simulink model "Sim_PIControl_PC"  (R2025b)
settings: Solver=VariableStepAuto  StartTime=0.0  StopTime=3  FixedStep=Ts  RelTol=1e-3
values from neighbouring files (symbols this model uses):
  Cf = Cf_values(k)    [Init_OSQP_PC.m]    (also in PC_PIControl.m = 1.2e-05)
  Ki_if = (sqrt(5) - 2)*Ki*wci^2    [PC_PIControl.m]
  Ki_vc = (sqrt(5) - 2)*Kv*wcv^2    [PC_PIControl.m]
  kP = ((2*pi*50.5) - (2*pi*49.5))/(2*10e3)    (= 0.000314159265359)    [PC_PIControl.m]
  Kp_if = (sqrt(2)*sqrt(sqrt(5) - 2))*Ki*wci    [PC_PIControl.m]
  Kp_vc = (sqrt(2)*sqrt(sqrt(5) - 2))*Kv*wcv    [PC_PIControl.m]
  kQ = (1.05*Vb - 0.95*Vb)/(10e3)    [PC_PIControl.m]
  Lf = Lf_values(k)    [Init_OSQP_PC.m]    (also in PC_PIControl.m = 0.005)
  Ts = 1/fs    (= 0.0002)    [Init_OSQP_PC.m]    (also in PC_PIControl.m)
  Vb = Vdc*(sqrt(3)/3)/1.15    [Init_OSQP_PC.m]    (also in PC_PIControl.m)
  wb = 2*pi*f    (= 314.159265359)    [Init_OSQP_PC.m]    (also in PC_PIControl.m)
  wc = 2*pi*10    (= 62.8318530718)    [PC_PIControl.m]
undefined symbols (not defined in the file or in its folder): plecs
settings Model: Creator=ASUS-PC  LastModifiedBy=dfigueroa
settings SolverCC: AllowMultiTaskInputOutput=on
settings DebuggingCC: IntegerOverflowMsg=error  ParameterPrecisionLossMsg=error  UnderSpecifiedDimensionMsg=warning
settings RTWCC: GPUComputeCapability=3.5

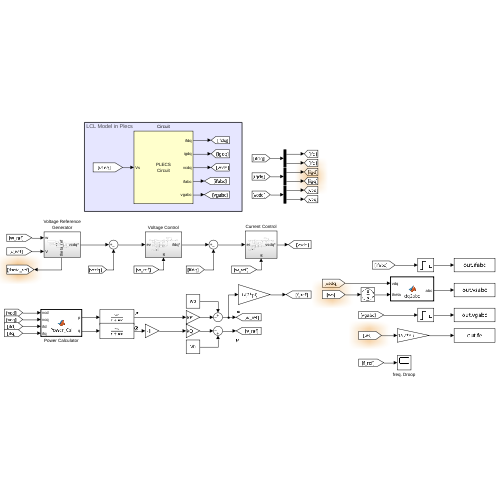
[thumbnail: Simulink's stored preview of the top-level diagram]
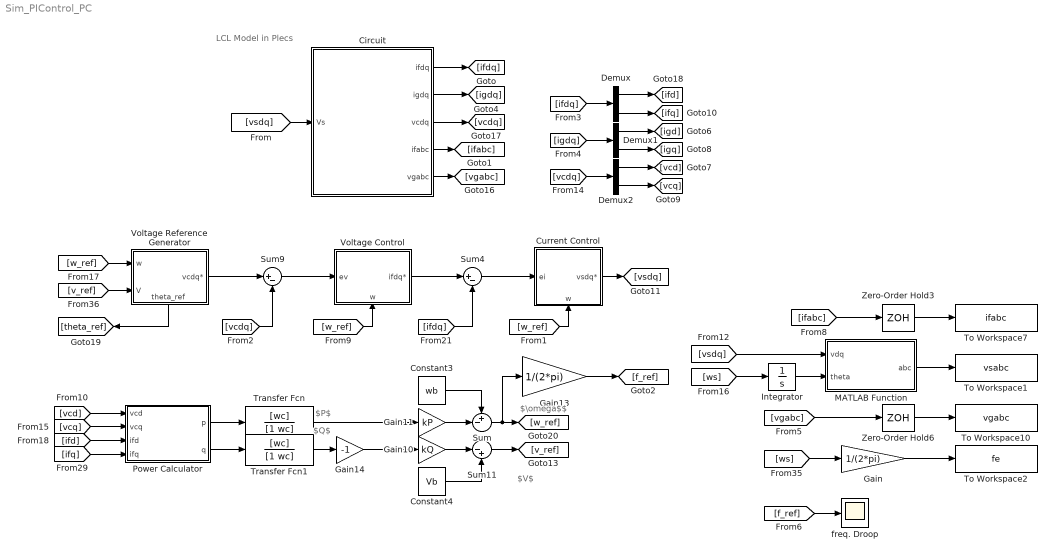
== system Sim_PIControl_PC ==
  note: $\omega$$
  note: LCL Model in Plecs
  note: $V$
  note: $P$
  note: $Q$
  Circuit : Subsystem  LoadFcn=plecs('sl', 200);  InitFcn=plecs('sl', 214);  StartFcn=plecs('sl', 208);  StopFcn=plecs('sl', 209);  mask(PlecsCircuit){PLECSData=<binary blob, 10232 chars, not shown>}
      mask prompts: PLECSData "PLECS Data (Do not delete or modify!)"
      mask init:
      | % PLACE CUSTOM INITIALIZATIONS ABOVE
      | % DO NOT REMOVE
      | plecs('sl', 215);
      | % DO NOT REMOVE
      settings: CopyFcn=plecs('sl', 203);  DeleteFcn=plecs('sl', 205);  UndoDeleteFcn=plecs('sl', 206);  PreSaveFcn=plecs('sl', 211);  PostSaveFcn=plecs('sl', 201);  NameChangeFcn=plecs('sl', 210);  DestroyFcn=plecs('sl', 207);  PreCopyFcn=plecs('sl', 216);  OpenFcn=plecs('sl', 202);  ErrorFcn=plerrorfcn
      mask Help: eval('plecs(''help'', ''qthelp:///creatingacircuit.html'')')
      mask Display: disp('PLECS\nCircuit')
  Constant3 : Constant  Value=wb
  Constant4 : Constant  Value=Vb
  Current Control : Subsystem
      settings: PortSchema="{\"entries\":[{\"content\":{\"sides\":[{\"content\":{\"connectorIds\":[\"In1\"]},\"type\":\"ConnectorPlacement.EquallySpacedRectSide\",\"uuid\":\"15de3949-f64d-4365-a71a-b55d33a0652a\"},{\"content\":{\"connectorIds\":[\"Out1\"],\"side\":\"RIGHT\"},\"type\":\"ConnectorPlacement.EquallySpacedRectSide\",\"uuid\":\"5304f75d-1e45-448d-a7e7-0abd1c4a85d7\"},{\"content\":{\"side\":\"TOP\"},\"type\":\"ConnectorPlacement.EquallySpacedRectSide\",\"uuid\":\"10b46e03-c30b-42fe-844b-139720435cf3\"},{\"content\":{\"connectorIds\":[\"In2\"],\"side\":\"BOTTOM\"},\"type\":\"ConnectorPlacement.EquallySpacedRectSide\",\"uuid\":\"b1e5226e-e07e-42fd-8e80-f79eeedd3ce4\"}]},\"type\":\"ConnectorPlacement.EquallySpacedConnector\",\"uuid\":\"fe8a93e2-75ca-4241-a8e5-189ba102a419\"}],\"packageUris\":[\"http://schema.mathworks.com/mf0/Connector/R2020b\"],\"version\":\"1.0\"}"
  Demux : Demux  Outputs=2
  Demux1 : Demux  Outputs=2
  Demux2 : Demux  Outputs=2
  Gain : Gain  Gain=1/(2*pi)
  Gain10 : Gain  Gain=kQ
  Gain11 : Gain  Gain=kP
  Gain13 : Gain  Gain=1/(2*pi)
  Gain14 : Gain  Gain=-1
  Integrator : Integrator  WrapState=on
  MATLAB Function : MATLAB Function  TreatAsAtomicUnit=on
  Power Calculator : MATLAB Function  TreatAsAtomicUnit=on
  Sum : Sum  Inputs=+-|
  Sum11 : Sum  Inputs=|-+
  Sum4 : Sum  Inputs=|+-
  Sum9 : Sum  Inputs=|+-
  To Workspace1 : ToWorkspace  VariableName=vsabc  SaveFormat=Structure With Time  SampleTime=Ts
  To Workspace10 : ToWorkspace  VariableName=vgabc  SaveFormat=Structure With Time  SampleTime=Ts
  To Workspace2 : ToWorkspace  VariableName=fe  SaveFormat=Structure With Time  SampleTime=Ts
  To Workspace7 : ToWorkspace  VariableName=ifabc  SaveFormat=Structure With Time  SampleTime=Ts
  Transfer Fcn : TransferFcn  Numerator=[wc]  Denominator=[1 wc]
  Transfer Fcn1 : TransferFcn  Numerator=[wc]  Denominator=[1 wc]
  Voltage Control : Subsystem
      settings: PortSchema="{\"entries\":[{\"content\":{\"sides\":[{\"content\":{\"connectorIds\":[\"In1\"]},\"type\":\"ConnectorPlacement.EquallySpacedRectSide\",\"uuid\":\"17694daf-e143-4e65-9b5e-1361fea51640\"},{\"content\":{\"connectorIds\":[\"Out1\"],\"side\":\"RIGHT\"},\"type\":\"ConnectorPlacement.EquallySpacedRectSide\",\"uuid\":\"ae099be1-6c63-48da-a018-cc27e2552eee\"},{\"content\":{\"side\":\"TOP\"},\"type\":\"ConnectorPlacement.EquallySpacedRectSide\",\"uuid\":\"be7d7428-f416-4c9d-8f40-1acc1e97d54d\"},{\"content\":{\"connectorIds\":[\"In2\"],\"side\":\"BOTTOM\"},\"type\":\"ConnectorPlacement.EquallySpacedRectSide\",\"uuid\":\"aed40d46-5854-41d6-a016-6ed5efe903e2\"}]},\"type\":\"ConnectorPlacement.EquallySpacedConnector\",\"uuid\":\"c5f51056-7a41-44d7-9f07-337f09c5458b\"}],\"packageUris\":[\"http://schema.mathworks.com/mf0/Connector/R2020b\"],\"version\":\"1.0\"}"
  Voltage Reference Generator : Subsystem
      settings: PortSchema="{\"entries\":[{\"content\":{\"sides\":[{\"content\":{\"connectorIds\":[\"In1\",\"In2\"]},\"type\":\"ConnectorPlacement.EquallySpacedRectSide\",\"uuid\":\"b26fa032-6e4d-44d9-b402-3e4f33c2239a\"},{\"content\":{\"connectorIds\":[\"Out1\"],\"side\":\"RIGHT\"},\"type\":\"ConnectorPlacement.EquallySpacedRectSide\",\"uuid\":\"fe4c0e2a-2db0-49b2-98ed-3d548f61cfff\"},{\"content\":{\"side\":\"TOP\"},\"type\":\"ConnectorPlacement.EquallySpacedRectSide\",\"uuid\":\"e31f001e-f282-4750-9f26-9a12e3ce4d4f\"},{\"content\":{\"connectorIds\":[\"Out2\"],\"side\":\"BOTTOM\"},\"type\":\"ConnectorPlacement.EquallySpacedRectSide\",\"uuid\":\"8214a013-4473-4dc7-97ac-10353f010234\"}]},\"type\":\"ConnectorPlacement.EquallySpacedConnector\",\"uuid\":\"06fb1ff6-6ff9-4330-922e-5349c8b7d67c\"}],\"packageUris\":[\"http://schema.mathworks.com/mf0/Connector/R2020b\"],\"version\":\"1.0\"}"
  Zero-Order Hold3 : ZeroOrderHold  SampleTime=Ts
  Zero-Order Hold6 : ZeroOrderHold  SampleTime=Ts
  freq. Droop : Scope
      settings: ActiveDisplayYMinimum=49.9993242494902  ActiveDisplayYMaximum=50.001983465796577
  wires:
  Circuit/5(vgabc) -> [vgabc]
  [vsdq] -> Circuit/1(Vs)
  Circuit/4(ifabc) -> [ifabc]
  Demux1/2 -> [igq]
  Demux/1 -> [ifd]
  Demux2/2 -> [vcq]
  Demux1/1 -> [igd]
  Demux2/1 -> [vcd]
  Demux/2 -> [ifq]
  Gain/1 -> To Workspace2/1
  Zero-Order Hold3/1 -> To Workspace7/1
  Integrator/1 -> MATLAB Function/2(theta)
  [ifabc] -> Zero-Order Hold3/1
  [vgabc] -> Zero-Order Hold6/1
  MATLAB Function/1(abc) -> To Workspace1/1
  Zero-Order Hold6/1 -> To Workspace10/1
  [ws] -> Integrator/1
  [vsdq] -> MATLAB Function/1(vdq)
  [ws] -> Gain/1
  [ifdq] -> Sum4/2
  Circuit/1(ifdq) -> [ifdq]
  Circuit/2(igdq) -> [igdq]
  Circuit/3(vcdq) -> [vcdq]
  [ifdq] -> Demux/1
  [igdq] -> Demux1/1
  [vcdq] -> Demux2/1
  [vcdq] -> Sum9/2
  [vcd] -> Power Calculator/1(vcd)
  [vcq] -> Power Calculator/2(vcq)
  [ifd] -> Power Calculator/3(ifd)
  [ifq] -> Power Calculator/4(ifq)
  Power Calculator/1(p) -> Transfer Fcn/1
  Power Calculator/2(q) -> Transfer Fcn1/1
  Constant4/1 -> Sum11/2
  [w_ref] -> Voltage Control/2(w)
  Sum11/1 -> [v_ref]
  Sum/1 -> [w_ref], Gain13/1
  Constant3/1 -> Sum/1
  Gain11/1 -> Sum/2
  Gain10/1 -> Sum11/1
  Transfer Fcn/1 -> Gain11/1
  Transfer Fcn1/1 -> Gain14/1
  Gain14/1 -> Gain10/1
  Sum9/1 -> Voltage Control/1(ev)
  Voltage Control/1(ifdq*) -> Sum4/1
  Sum4/1 -> Current Control/1(ei)
  Current Control/1(vsdq*) -> [vsdq]
  [w_ref] -> Current Control/2(w)
  [w_ref] -> Voltage Reference Generator/1(w)
  [v_ref] -> Voltage Reference Generator/2(V)
  Voltage Reference Generator/1(vcdq*) -> Sum9/1
  Voltage Reference Generator/2(theta_ref) -> [theta_ref]
  Gain13/1 -> [f_ref]
  [f_ref] -> freq. Droop/1

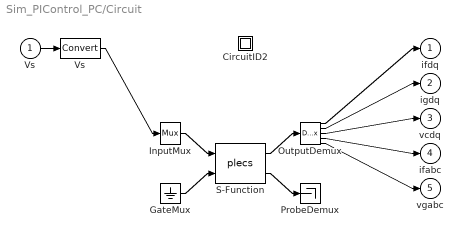
== system Sim_PIControl_PC/Circuit ==
  Vs : Inport  PortDimensions=2
  " CircuitID2 " : Subsystem
  " GateMux " : Ground
  " InputMux " : Mux  Inputs=[ 2 ]
  " OutputDemux " : Demux  Outputs=[ 2 2 2 3 3 ]
  " ProbeDemux " : Terminator
  " S-Function " : S-Function  FunctionName=plecs  SFunctionDeploymentMode=off  EnableBusSupport=off
  " Vs " : DataTypeConversion
  ifdq : Outport  PortDimensions=2
  igdq : Outport  Port=2  PortDimensions=2
  vcdq : Outport  Port=3  PortDimensions=2
  ifabc : Outport  Port=4  PortDimensions=3
  vgabc : Outport  Port=5  PortDimensions=3
  wires:
  " InputMux "/1 -> " S-Function "/1
  " GateMux "/1 -> " S-Function "/2
  " S-Function "/1 -> " OutputDemux "/1
  " S-Function "/2 -> " ProbeDemux "/1
  Vs/1 -> " Vs "/1
  " Vs "/1 -> " InputMux "/1
  " OutputDemux "/1 -> ifdq/1
  " OutputDemux "/2 -> igdq/1
  " OutputDemux "/3 -> vcdq/1
  " OutputDemux "/4 -> ifabc/1
  " OutputDemux "/5 -> vgabc/1

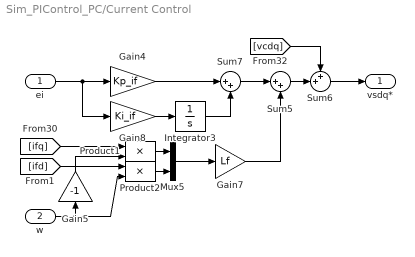
== system Sim_PIControl_PC/Current Control ==
  ei : Inport
  w : Inport  Port=2
  Gain4 : Gain  Gain=Kp_if
  Gain5 : Gain  Gain=-1
  Gain7 : Gain  Gain=Lf
  Gain8 : Gain  Gain=Ki_if
  Integrator3 : Integrator
  Mux5 : Mux  Inputs=2
  Product1 : Product
  Product2 : Product
  Sum5 : Sum  Inputs=|++
  Sum6 : Sum  Inputs=++|
  Sum7 : Sum  Inputs=|++
  vsdq* : Outport
  wires:
  Product1/1 -> Mux5/1
  Mux5/1 -> Gain7/1
  Gain8/1 -> Integrator3/1
  ei/1 -> Gain8/1, Gain4/1
  [ifq] -> Product1/1
  Sum6/1 -> vsdq*/1
  Sum5/1 -> Sum6/2
  Gain4/1 -> Sum7/1
  Integrator3/1 -> Sum7/2
  [ifd] -> Product2/1
  Gain7/1 -> Sum5/2
  Sum7/1 -> Sum5/1
  Product2/1 -> Mux5/2
  Gain5/1 -> Product1/2
  [vcdq] -> Sum6/1
  w/1 -> Gain5/1, Product2/2

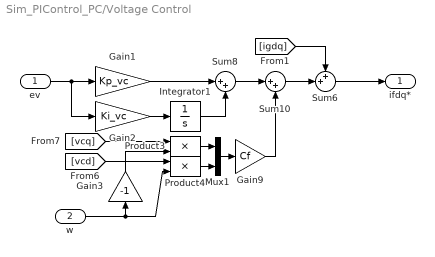
== system Sim_PIControl_PC/Voltage Control ==
  ev : Inport
  w : Inport  Port=2
  Gain1 : Gain  Gain=Kp_vc
  Gain2 : Gain  Gain=Ki_vc
  Gain3 : Gain  Gain=-1
  Gain9 : Gain  Gain=Cf
  Integrator1 : Integrator
  Mux1 : Mux  Inputs=2
  Product3 : Product
  Product4 : Product
  Sum10 : Sum  Inputs=|++
  Sum6 : Sum  Inputs=++|
  Sum8 : Sum  Inputs=|++
  ifdq* : Outport
  wires:
  Gain9/1 -> Sum10/2
  Sum10/1 -> Sum6/2
  w/1 -> Product4/2, Gain3/1
  Gain1/1 -> Sum8/1
  Integrator1/1 -> Sum8/2
  [vcq] -> Product3/1
  Gain2/1 -> Integrator1/1
  Mux1/1 -> Gain9/1
  Sum8/1 -> Sum10/1
  [vcd] -> Product4/1
  Product4/1 -> Mux1/2
  Gain3/1 -> Product3/2
  ev/1 -> Gain2/1, Gain1/1
  Product3/1 -> Mux1/1
  Sum6/1 -> ifdq*/1
  [igdq] -> Sum6/1

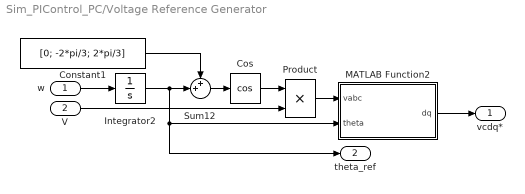
== system Sim_PIControl_PC/Voltage Reference Generator ==
  w : Inport
  V : Inport  Port=2
  Constant1 : Constant  Value=[0; -2*pi/3; 2*pi/3]
  Cos : Trigonometry  Operator=cos
  Integrator2 : Integrator
  MATLAB Function2 : MATLAB Function  TreatAsAtomicUnit=on
  Product : Product
  Sum12 : Sum  Inputs=++|
  vcdq* : Outport
  theta_ref : Outport  Port=2
  wires:
  Product/1 -> MATLAB Function2/1(vabc)
  Cos/1 -> Product/1
  Sum12/1 -> Cos/1
  Constant1/1 -> Sum12/1
  MATLAB Function2/1(dq) -> vcdq*/1
  Integrator2/1 -> Sum12/2, theta_ref/1, MATLAB Function2/2(theta)
  w/1 -> Integrator2/1
  V/1 -> Product/2

== system Sim_PIControl_PC/Circuit/ CircuitID2  ==

== matlab function Sim_PIControl_PC/MATLAB Function ==
  data: vdq input; abc output; theta input
function abc = dq2abc(vdq,theta)
    T = [sin(theta)        -sin(theta)        ;
         cos(theta-2*pi/3) -sin(theta-2*pi/3) ;
         cos(theta+2*pi/3) -sin(theta+2*pi/3)];
    abc = T*vdq;

== matlab function Sim_PIControl_PC/Power Calculator ==
  data: vcd input; p output; vcq input; ifd input; ifq input; q output
function [p,q] = Power_Cal(vcd,vcq,ifd,ifq)
    p = (3/2)*(vcd*ifd + vcq*ifq);
    q = (3/2)*(vcq*ifd - vcd*ifq);

== matlab function Sim_PIControl_PC/Voltage Reference Generator/MATLAB Function2 ==
  data: vabc input; dq output; theta input
function dq = abc2dq(vabc,theta)
    T = [ cos(theta)   cos(theta-2*pi/3)   cos(theta+2*pi/3) ;
         -sin(theta)  -sin(theta-2*pi/3)  -sin(theta+2*pi/3)];
    dq = (2/3)*T*vabc;
